simulink model "MCC"  (R2017b)
settings: Solver=ode15s  StartTime=0.0  StopTime=0.5  RelTol=1e-3
InitFcn:
  | TD2_config
values from neighbouring files (symbols this model uses):
  b = 8.5E-3    (= 0.0085)    [TD2_config.m]
  Cr = 0    [TD2_config.m]
  J = 0.28    [TD2_config.m]
  K = 0.5093    [TD2_config.m]
  Kd = 0.028    [TD2_config.m]
  Ki = 28    [TD2_config.m]
  Kp = 3    [TD2_config.m]
  Kpos = 6    [TD2_config.m]
  L = 1.6E-3    (= 0.0016)    [TD2_config.m]
  R = 0.13    [TD2_config.m]
libraries: simulink x7
settings Model: Creator=TABLE 6  LastModifiedBy=TP-EO-5

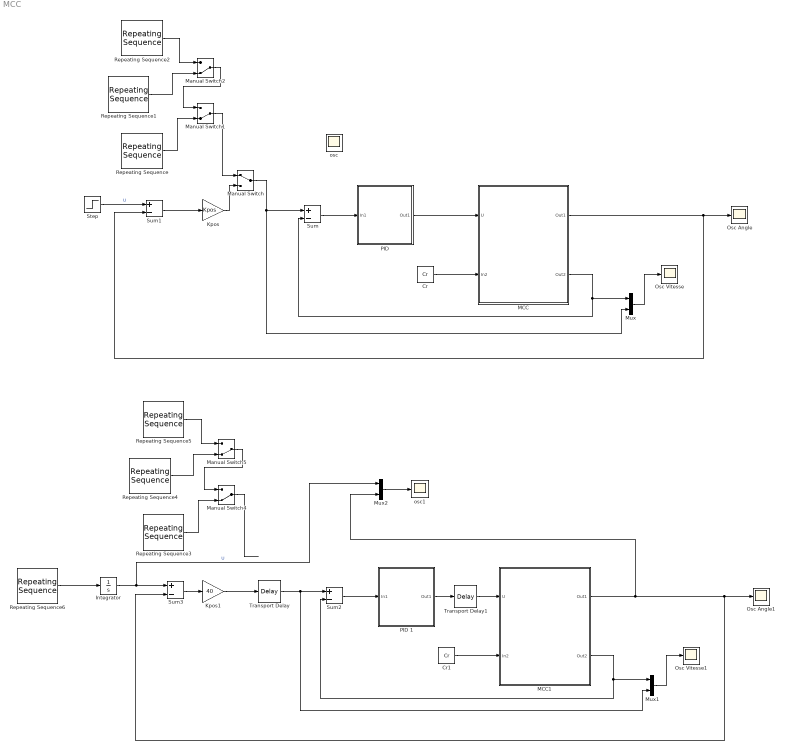
== system MCC ==
  Cr : Constant  Value=Cr
  Cr1 : Constant  Value=Cr
  Integrator : Integrator
  Kpos : Gain  Gain=Kpos
  Kpos1 : Gain  Gain=40
  MCC : Subsystem
  MCC1 : Subsystem
  Manual Switch : ManualSwitch
  Manual Switch{1..2,4..5} (4 alike) : ManualSwitch  CurrentSetting=0
  Mux : Mux  Inputs=2
  Mux1 : Mux  Inputs=2
  Mux2 : Mux  Inputs=2
  Osc Angle : Scope
  Osc Angle1 : Scope
  Osc Vitesse : Scope
  Osc Vitesse1 : Scope
  "PID " : Subsystem
  PID 1 : Subsystem
  Repeating Sequence : simulink/Sources/Repeating Sequence  rep_seq_t=[0 0.1 0.2 0.3 1]  rep_seq_y=[0 50 50 0 0]
  Repeating Sequence1 : simulink/Sources/Repeating Sequence  rep_seq_t=[0 0.049 0.05 0.25 0.251 0.3 1]  rep_seq_y=[0 0 50 50 0 0 0]
  Repeating Sequence2 : simulink/Sources/Repeating Sequence  rep_seq_t=[0 0.15 0.3 1]  rep_seq_y=[0 67 0 0]
  Repeating Sequence3 : simulink/Sources/Repeating Sequence  rep_seq_t=[0 0.1 0.2 0.3 1]  rep_seq_y=[0 50 50 0 0]
  Repeating Sequence4 : simulink/Sources/Repeating Sequence  rep_seq_t=[0 0.049 0.05 0.25 0.251 0.3 1]  rep_seq_y=[0 0 50 50 0 0 0]
  Repeating Sequence5 : simulink/Sources/Repeating Sequence  rep_seq_t=[0 0.15 0.3 1]  rep_seq_y=[0 67 0 0]
  Repeating Sequence6 : simulink/Sources/Repeating Sequence  rep_seq_t=[0 0.1 0.2 0.3 1]  rep_seq_y=[0 50 50 0 0]
  Step : Step  Time=0  SampleTime=0
  Sum{,1..3} (4 alike) : Sum  Inputs=+-
  Transport Delay : TransportDelay  DelayTime=0.02
  Transport Delay1 : TransportDelay  DelayTime=0
  osc : Scope
  osc1 : Scope
  wires:
  Cr/1 -> MCC/2(In2)
  MCC/1(Out1) -> Sum1/2, Osc Angle/1
  MCC/2(Out2) -> Mux/1, Sum/2
  Sum/1 -> "PID "/1(In1)
  "PID "/1(Out1) -> MCC/1(U)
  Step/1 -> Sum1/1  "U"
  Sum1/1 -> Kpos/1
  Kpos/1 -> Manual Switch/2
  Manual Switch/1 -> Sum/1, Mux/2
  Mux/1 -> Osc Vitesse/1
  Repeating Sequence1/1 -> Manual Switch2/2
  Manual Switch1/1 -> Manual Switch/1
  Repeating Sequence/1 -> Manual Switch1/2
  Manual Switch2/1 -> Manual Switch1/1
  Repeating Sequence2/1 -> Manual Switch2/1
  Mux1/1 -> Osc Vitesse1/1
  Sum3/1 -> Kpos1/1
  Repeating Sequence4/1 -> Manual Switch5/2
  Integrator/1 -> Mux2/1, Sum3/1  "U"
  Repeating Sequence5/1 -> Manual Switch5/1
  Manual Switch5/1 -> Manual Switch4/1
  Manual Switch4/1 -> ?
  Repeating Sequence3/1 -> Manual Switch4/2
  PID 1/1(Out1) -> Transport Delay1/1
  MCC1/2(Out2) -> Mux1/1, Sum2/2
  Sum2/1 -> PID 1/1(In1)
  MCC1/1(Out1) -> Mux2/2, Sum3/2, Osc Angle1/1
  Cr1/1 -> MCC1/2(In2)
  Repeating Sequence6/1 -> Integrator/1
  Mux2/1 -> osc1/1
  Transport Delay/1 -> Mux1/2, Sum2/1
  Kpos1/1 -> Transport Delay/1
  Transport Delay1/1 -> MCC1/1(U)

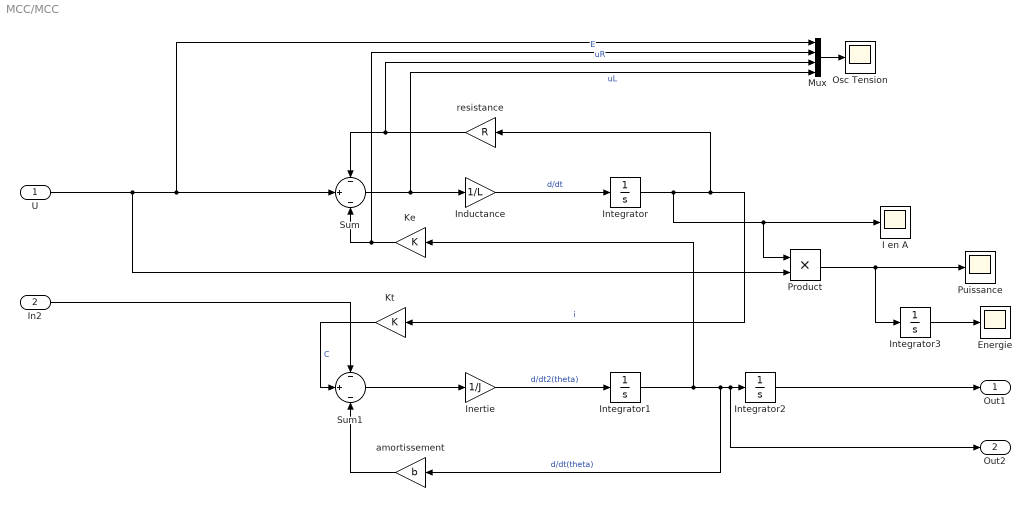
== system MCC/MCC ==
  U : Inport
  In2 : Inport  Port=2
  "Energie " : Scope
  I en A : Scope
  Inductance : Gain  Gain=1/L
  Inertie : Gain  Gain=1/J
  Integrator{,1..3} (4 alike) : Integrator
  Ke : Gain  Gain=K
  Kt : Gain  Gain=K
  Mux : Mux
  Osc Tension : Scope
  Product : Product
  Puissance : Scope
  Sum : Sum  Inputs=-|+|-
  Sum1 : Sum  Inputs=-|+|-
  amortissement : Gain  Gain=b
  resistance : Gain  Gain=R
  Out1 : Outport
  Out2 : Outport  Port=2
  wires:
  resistance/1 -> Mux/3, Sum/1  "uR"
  Sum/1 -> Mux/4, Inductance/1  "uL"
  Inductance/1 -> Integrator/1  "d/dt"
  Inertie/1 -> Integrator1/1  "d/dt2(theta)"
  Sum1/1 -> Inertie/1
  Mux/1 -> Osc Tension/1
  Integrator1/1 -> Ke/1, amortissement/1, Out2/1, Integrator2/1  "d/dt(theta)"
  U/1 -> Product/2, Mux/1, Sum/2
  Integrator2/1 -> Out1/1
  Integrator/1 -> Product/1, I en A/1, resistance/1, Kt/1  "i"
  In2/1 -> Sum1/1
  amortissement/1 -> Sum1/3
  Ke/1 -> Mux/2, Sum/3  "E"
  Kt/1 -> Sum1/2  "C"
  Product/1 -> Integrator3/1, Puissance/1
  Integrator3/1 -> "Energie "/1

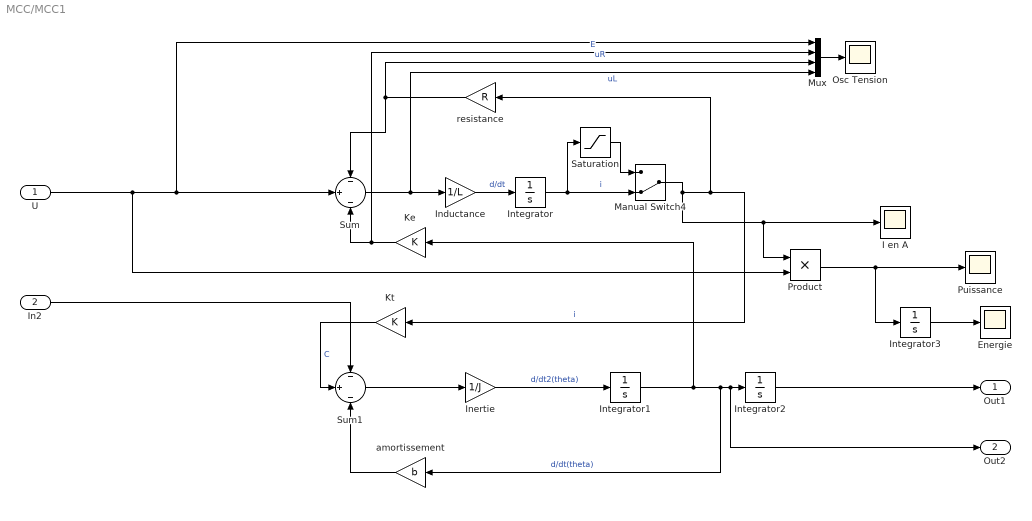
== system MCC/MCC1 ==
  U : Inport
  In2 : Inport  Port=2
  "Energie " : Scope
  I en A : Scope
  Inductance : Gain  Gain=1/L
  Inertie : Gain  Gain=1/J
  Integrator{,1..3} (4 alike) : Integrator
  Ke : Gain  Gain=K
  Kt : Gain  Gain=K
  Manual Switch4 : ManualSwitch  CurrentSetting=0
  Mux : Mux
  Osc Tension : Scope
  Product : Product
  Puissance : Scope
  Saturation : Saturate  UpperLimit=300  LowerLimit=-300
  Sum : Sum  Inputs=-|+|-
  Sum1 : Sum  Inputs=-|+|-
  amortissement : Gain  Gain=b
  resistance : Gain  Gain=R
  Out1 : Outport
  Out2 : Outport  Port=2
  wires:
  resistance/1 -> Sum/1, Mux/3  "uR"
  Sum/1 -> Mux/4, Inductance/1  "uL"
  Inductance/1 -> Integrator/1  "d/dt"
  Inertie/1 -> Integrator1/1  "d/dt2(theta)"
  Sum1/1 -> Inertie/1
  Mux/1 -> Osc Tension/1
  Integrator1/1 -> Ke/1, amortissement/1, Out2/1, Integrator2/1  "d/dt(theta)"
  U/1 -> Product/2, Mux/1, Sum/2
  Integrator2/1 -> Out1/1
  Manual Switch4/1 -> Product/1, I en A/1, resistance/1, Kt/1  "i"
  In2/1 -> Sum1/1
  amortissement/1 -> Sum1/3
  Ke/1 -> Mux/2, Sum/3  "E"
  Kt/1 -> Sum1/2  "C"
  Product/1 -> Integrator3/1, Puissance/1
  Integrator3/1 -> "Energie "/1
  Integrator/1 -> Saturation/1, Manual Switch4/2  "i"
  Saturation/1 -> Manual Switch4/1

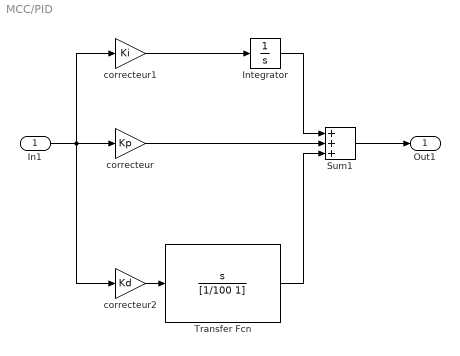
== system MCC/PID  ==
  In1 : Inport
  Integrator : Integrator
  Sum1 : Sum  Inputs=+++
  Transfer Fcn : TransferFcn  Numerator=[1 0]  Denominator=[1/100 1]
  correcteur : Gain  Gain=Kp
  correcteur1 : Gain  Gain=Ki
  correcteur2 : Gain  Gain=Kd
  Out1 : Outport
  wires:
  Sum1/1 -> Out1/1
  In1/1 -> correcteur2/1, correcteur1/1, correcteur/1
  correcteur1/1 -> Integrator/1
  correcteur/1 -> Sum1/2
  Transfer Fcn/1 -> Sum1/3
  Integrator/1 -> Sum1/1
  correcteur2/1 -> Transfer Fcn/1

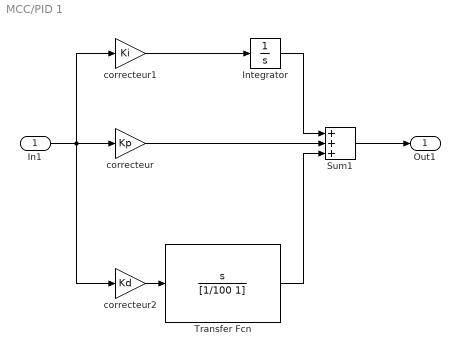
== system MCC/PID 1 ==
  In1 : Inport
  Integrator : Integrator
  Sum1 : Sum  Inputs=+++
  Transfer Fcn : TransferFcn  Numerator=[1 0]  Denominator=[1/100 1]
  correcteur : Gain  Gain=Kp
  correcteur1 : Gain  Gain=Ki
  correcteur2 : Gain  Gain=Kd
  Out1 : Outport
  wires:
  Sum1/1 -> Out1/1
  In1/1 -> correcteur2/1, correcteur1/1, correcteur/1
  correcteur1/1 -> Integrator/1
  correcteur/1 -> Sum1/2
  Transfer Fcn/1 -> Sum1/3
  Integrator/1 -> Sum1/1
  correcteur2/1 -> Transfer Fcn/1
